simulink model "Triangular_Signal"  (R2023b)
settings: Solver=VariableStepAuto  StartTime=0.0  StopTime=10.0  RelTol=1e-3
settings Model: Creator=hkurt  LastModifiedBy=hkurt

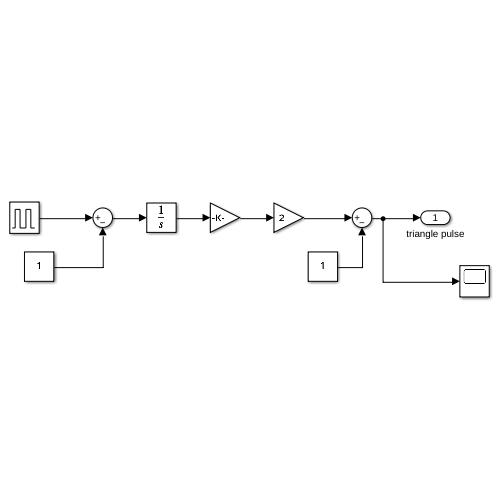
[thumbnail: Simulink's stored preview of the top-level diagram]
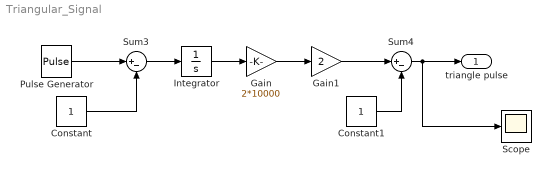
== system Triangular_Signal ==
  Constant : Constant
  Constant1 : Constant
  Gain : Gain  Gain=2*10000
  Gain1 : Gain  Gain=2
  Integrator : Integrator
  Pulse Generator : DiscretePulseGenerator  PulseType=Time based  Amplitude=2  Period=1/10000  PulseWidth=50
  Scope : Scope
  Sum3 : Sum  Inputs=|+-
  Sum4 : Sum  Inputs=|+-
  triangle pulse : Outport
  wires:
  Sum3/1 -> Integrator/1
  Pulse Generator/1 -> Sum3/1
  Constant1/1 -> Sum4/2
  Gain1/1 -> Sum4/1
  Constant/1 -> Sum3/2
  Gain/1 -> Gain1/1
  Sum4/1 -> Scope/1, triangle pulse/1
  Integrator/1 -> Gain/1
